simulink model "W01_OpenClosed"  (R2024b)
settings: Solver=ode45  StartTime=0.0  StopTime=t_end  MaxStep=0.01  RelTol=1e-3
PreLoadFcn:
  | % W01_OpenClosed 기본 파라미터 (모델을 열 때 자동 실행)
  | % 이미 워크스페이스에 값이 있으면 그대로 두고, 없을 때만 채웁니다.
  | defs = { 'm',1 ; 'b',0.2 ; 'k',1 ; 'r',1 ; 'd',0.5 ; 't_d',40 ;
  |          't_end',100 ; 'K',9 ; 'Kff',1 ; 'Kr',10/9 };
  | for ii = 1:size(defs,1)
  |     if ~evalin('base', sprintf('exist(''%s'',''var'')', defs{ii,1}))
  |         assignin('base', defs{ii,1}, defs{ii,2});
  |     end
  | end
  | clear defs ii
values from neighbouring files (symbols this model uses):
  b = p.b    [W01_03_run_simulink.m]
  d = 0.5    [W01_01_open_vs_closed.m]    (also in W01_03_run_simulink.m)
  K = 9    [W01_01_open_vs_closed.m]    (also in W01_02_model_uncertainty.m; W01_03_run_simulink.m)
  k = p.k    [W01_03_run_simulink.m]
  Kff = 1 / dcgain(G)    [W01_01_open_vs_closed.m]    (also in W01_02_model_uncertainty.m = 1 / dcgain(G_design); W01_03_run_simulink.m)
  Kr = 1 / dcgain(T)    [W01_01_open_vs_closed.m]    (also in W01_02_model_uncertainty.m = 1 / dcgain(feedback(K*G_design, 1)); W01_03_run_simulink.m = 1 / dcgain(feedback(K*G, 1)))
  m = p.m    [W01_03_run_simulink.m]
  r = 1    [W01_01_open_vs_closed.m]    (also in W01_02_model_uncertainty.m; W01_03_run_simulink.m)
  t_d = 40    [W01_01_open_vs_closed.m]    (also in W01_03_run_simulink.m)
settings Model: Creator=admin  LastModifiedBy=wkyou

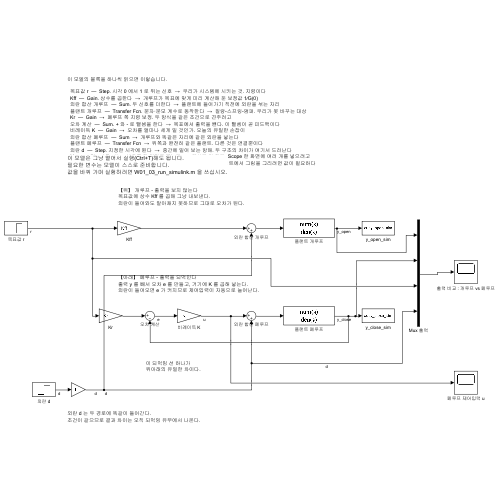
[thumbnail: Simulink's stored preview of the top-level diagram]
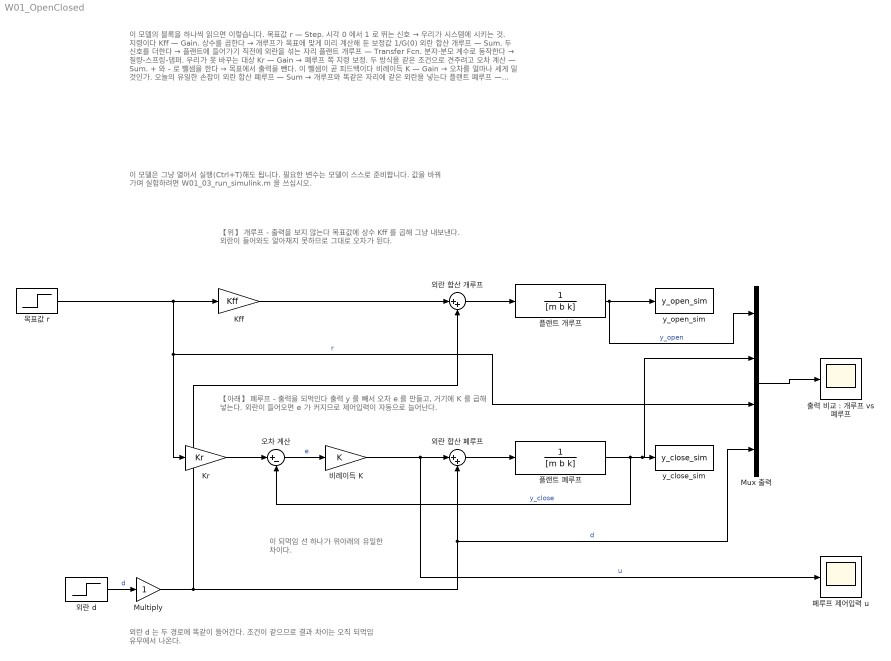
== system W01_OpenClosed ==
  note: 【위】 개루프 - 출력을 보지 않는다
      | 목표값에 상수 Kff 를 곱해 그냥 내보낸다.
      | 외란이 들어와도 알아채지 못하므로 그대로 오차가 된다.
  note: 【아래】 폐루프 - 출력을 되먹인다
      | 출력 y 를 빼서 오차 e 를 만들고, 거기에 K 를 곱해 넣는다.
      | 외란이 들어오면 e 가 커지므로 제어입력이 자동으로 늘어난다.
  note: 이 되먹임 선 하나가
      | 위아래의 유일한 차이다.
  note: 외란 d 는 두 경로에 똑같이 들어간다.
      | 조건이 같으므로 결과 차이는 오직 되먹임 유무에서 나온다.
  note: 이 모델은 그냥 열어서 실행(Ctrl+T)해도 됩니다.
      | 필요한 변수는 모델이 스스로 준비합니다.
      | 값을 바꿔 가며 실험하려면 W01_03_run_simulink.m 을 쓰십시오.
  note: 이 모델의 블록을 하나씩 읽으면 이렇습니다.
      |
      |   목표값 r  —  Step. 시각 0 에서 1 로 뛰는 신호  →  우리가 시스템에 시키는 것. 지령이다
      |   Kff  —  Gain. 상수를 곱한다  →  개루프가 목표에 맞게 미리 계산해 둔 보정값 1∕G(0)
      |   외란 합산 개루프  —  Sum. 두 신호를 더한다  →  플랜트에 들어가기 직전에 외란을 섞는 자리
      |   플랜트 개루프  —  Transfer Fcn. 분자·분모 계수로 동작한다  →  질량-스프링-댐퍼. 우리가 못 바꾸는 대상
      |   Kr  —  Gain  →  폐루프 쪽 지령 보정. 두 방식을 같은 조건으로 견주려고
      |   오차 계산  —  Sum. + 와 - 로 뺄셈을 한다  →  목표에서 출력을 뺀다. 이 뺄셈이 곧 피드백이다
      |   비례이득 K  —  Gain  →  오차를 얼마나 세게 밀 것인가. 오늘의 유일한 손잡이
      |   외란 합산 폐루프  —  Sum  →  개루프와 똑같은 자리에 같은 외란을 넣는다
      |   플랜트 폐루프  —  Transfer Fcn  →  위쪽과 완전히 같은 플랜트. 다른 것은 연결뿐이다
      |   외란 d  —  Step. 지정한 시각에 뛴다  →  중간에 밀어 보는 방해. 두 구조의 차이가 여기서 드러난다
      |   Mux  —  Signal Routing. 신호를 한 다발로 묶는다  →  계산은 안 한다. Scope 한 화면에 여러 개를 넣으려고
      |   To Workspace  —  신호를 MATLAB 작업공간으로 내보낸다  →  스크립트에서 그림을 그리려면 값이 필요하다
      |   Scope  —  신호를 그래프로 보여 준다  →  실행하면 자동으로 열린다
  Kff : Gain  Gain=Kff
  Kr : Gain  Gain=Kr
  Multiply : Gain
  Mux 출력 : Mux
  y_close_sim : ToWorkspace  VariableName=y_close_sim  SaveFormat=Timeseries  SampleTime=-1
  y_open_sim : ToWorkspace  VariableName=y_open_sim  SaveFormat=Timeseries  SampleTime=-1
  목표값 r : Step  Time=0  After=r  SampleTime=0
  비례이득 K : Gain  Gain=K
  오차 계산 : Sum  Inputs=|+-
  외란 d : Step  Time=t_d  After=d  SampleTime=0
  외란 합산 개루프 : Sum  Inputs=|++
  외란 합산 폐루프 : Sum  Inputs=|++
  "출력 비교 : 개루프 vs 폐루프" : Scope
  폐루프 제어입력 u : Scope
  플랜트 개루프 : TransferFcn  Denominator=[m b k]
  플랜트 폐루프 : TransferFcn  Denominator=[m b k]
  wires:
  목표값 r/1 -> Kr/1, Mux 출력/3, Kff/1  "r"
  Kff/1 -> 외란 합산 개루프/1
  외란 d/1 -> Multiply/1  "d"
  외란 합산 개루프/1 -> 플랜트 개루프/1
  플랜트 개루프/1 -> y_open_sim/1, Mux 출력/1  "y_open"
  Kr/1 -> 오차 계산/1
  오차 계산/1 -> 비례이득 K/1  "e"
  비례이득 K/1 -> 폐루프 제어입력 u/1, 외란 합산 폐루프/1  "u"
  외란 합산 폐루프/1 -> 플랜트 폐루프/1
  플랜트 폐루프/1 -> 오차 계산/2, y_close_sim/1, Mux 출력/2  "y_close"
  Mux 출력/1 -> "출력 비교 : 개루프 vs 폐루프"/1
  Multiply/1 -> 외란 합산 폐루프/2, Mux 출력/4, 외란 합산 개루프/2  "d"
